simulink model "rotElim"  (Simulink 8.4)
settings: Solver=ode45  StartTime=0.0  StopTime=10.0  RelTol=1e-3
settings Model: Creator=Alexey  LastModifiedBy=Dejan
settings DataIOCC: SignalLoggingSaveFormat=Dataset
settings OptimizationCC: InlineParams=on
settings DebuggingCC: FcnCallInpInsideContextMsg=EnableAllAsError
settings GRTTargetCC: CombineOutputUpdateFcns=on  GRTInterface=off

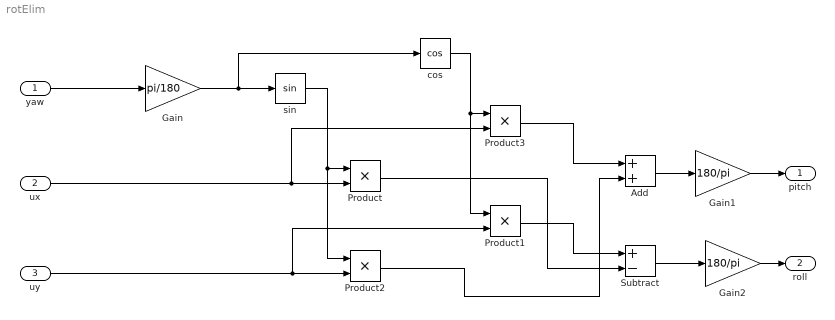
== system rotElim ==
  yaw : Inport
  ux : Inport  Port=2
  uy : Inport  Port=3
  Add : Sum
  Gain : Gain  Gain=pi/180
  Gain1 : Gain  Gain=180/pi
  Gain2 : Gain  Gain=180/pi
  Product{,1..3} (4 alike) : Product  RndMeth=Zero
  Subtract : Sum  Inputs=+-
  cos : Trigonometry  Operator=cos
  sin : Trigonometry
  pitch : Outport
  roll : Outport  Port=2
  wires:
  sin/1 -> Product2/1, Product/1
  cos/1 -> Product1/1, Product3/1
  Product1/1 -> Subtract/1
  Product2/1 -> Add/2
  Product3/1 -> Add/1
  Product/1 -> Subtract/2
  ux/1 -> Product3/2, Product/2
  uy/1 -> Product1/2, Product2/2
  Gain/1 -> cos/1, sin/1
  yaw/1 -> Gain/1
  Gain1/1 -> pitch/1
  Add/1 -> Gain1/1
  Gain2/1 -> roll/1
  Subtract/1 -> Gain2/1
